simulink model "PWM"  (R2024a)
settings: Solver=VariableStepAuto  StartTime=0.0  StopTime=T_end  RelTol=1e-3
values from neighbouring files (symbols this model uses):
  T_end = 0.1    [running_PWM_ver2.m]
  Ts = 0.000001    (= 1e-06)    [running_PWM_ver2.m]
libraries: simulink x1
settings Model: Creator=Design And Control  LastModifiedBy=jjw
settings DebuggingCC: UnderSpecifiedDimensionMsg=warning
settings SFSimCC: SimCustomHeaderCode="#include \"PWM.h\""  SimCustomInitializer=init(freq, duty);  SimUserSources=PWM.c  SimDebugExecutionForCustomCode=on

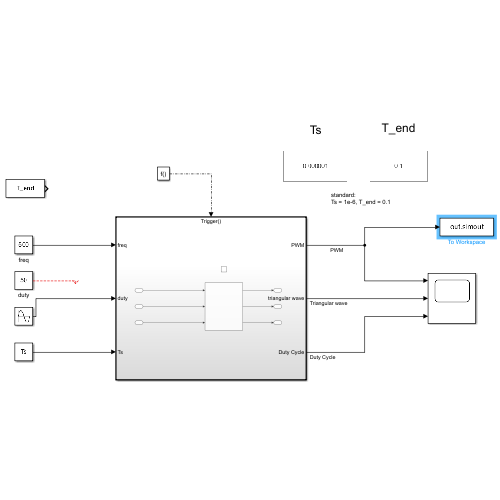
[thumbnail: Simulink's stored preview of the top-level diagram]
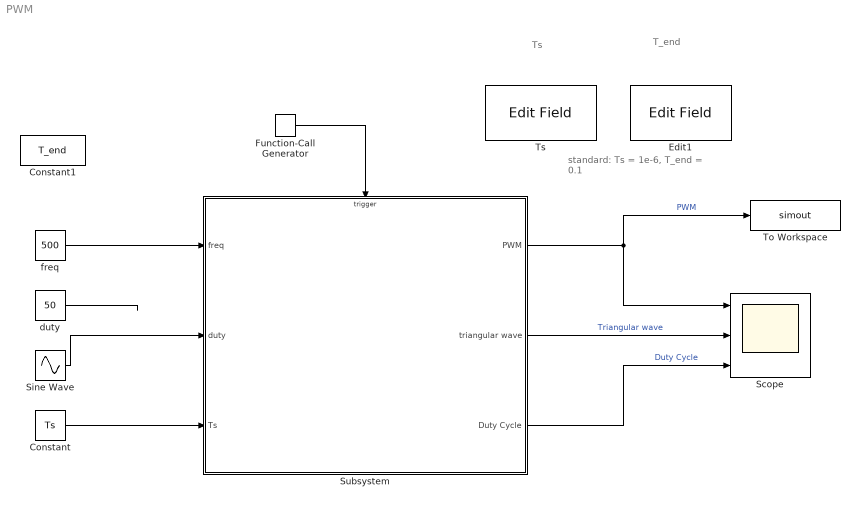
== system PWM ==
  note: standard:
      | Ts = 1e-6, T_end = 0.1
  note: Ts
  note: T_end
  Constant : Constant  Value=Ts
  Constant1 : Constant  Value=T_end
  Edit1 : EditField  LabelPosition=Hide  ShowInitialText=on  Alignment=Center
  Function-Call Generator : simulink/Ports & Subsystems/Function-Call Generator  sample_time=Ts  numberOfIterations=1  DisallowWideOutput=off
  Scope : Scope  NumInputPorts=3
  Sine Wave : Sin  Amplitude=50  Bias=50  Frequency=10*2*pi  SampleTime=0
  Subsystem : Subsystem
  To Workspace : ToWorkspace  VariableName=simout  SampleTime=-1
  Ts : EditField  LabelPosition=Hide  ShowInitialText=on  Alignment=Center
  duty : Constant  Value=50
  freq : Constant  Value=500
  wires:
  Sine Wave/1 -> Subsystem/2(duty)
  freq/1 -> Subsystem/1(freq)
  Subsystem/1(PWM) -> To Workspace/1, Scope/1  "PWM"
  Function-Call Generator/1 -> Subsystem/Trigger
  Subsystem/2(triangular wave) -> Scope/2  "Triangular wave"
  Subsystem/3(Duty Cycle) -> Scope/3  "Duty Cycle"
  Constant/1 -> Subsystem/3(Ts)
  duty/1 -> ?

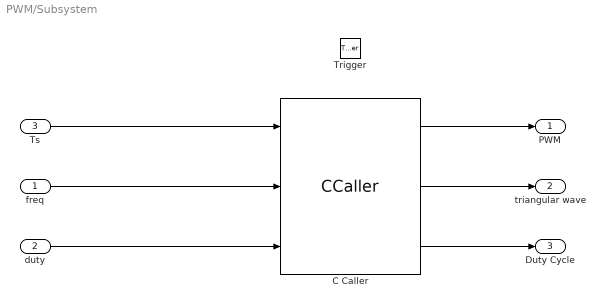
== system PWM/Subsystem ==
  freq : Inport
  duty : Inport  Port=2
  Ts : Inport  Port=3
  Trigger : TriggerPort  TriggerType=function-call  VariantControl=Variant  PortDimensions=1
  C Caller : CCaller  FunctionName=generatingPWM  PortSpecificationStruct="%)30     .    6 H   8    (     @         %    \"     8    !     0         %  0 \"0    $    _    07)G3F%M90  4&]R=$YA;64 4V-O<&4     26YD97@     5'EP90      4VEZ90      27-';&]B86P   X    P    !@    @    $          4    (     0    (    !         !   @!4<P  #@   #     &    \"     0         !0    @    !     @    $         $  \" %1S   .    .     8    (    !          %    \"     $    %     0         0  ...(+3186 chars)"
  PWM : Outport  OutDataTypeStr=double  Unit=1
  triangular wave : Outport  Port=2
  Duty Cycle : Outport  Port=3
  wires:
  duty/1 -> C Caller/3
  C Caller/1 -> PWM/1
  freq/1 -> C Caller/2
  C Caller/2 -> triangular wave/1
  C Caller/3 -> Duty Cycle/1
  Ts/1 -> C Caller/1
